simulink model "MPC_sim_noswitch"  (R2017b)
settings: Solver=VariableStepAuto  StartTime=0.0  StopTime=50  FixedStep=0.002  RelTol=1e-3
model workspace (MAT data in the model file):
  ref = Simulink.Parameter
  ref.DataType = 'double'
  ref.Dimensions = [0 0]
libraries: simulink x2, mpclib x1, dspmtrx3 x1
settings Model: Creator=pimwu  LastModifiedBy=pimwu
settings SolverCC: ZeroCrossAlgorithm=Adaptive
settings OptimizationCC: LifeSpan=inf
settings DebuggingCC: SFExecutionAtInitializationDiag=none
settings CodeAppCC: StateflowObjectComments=on

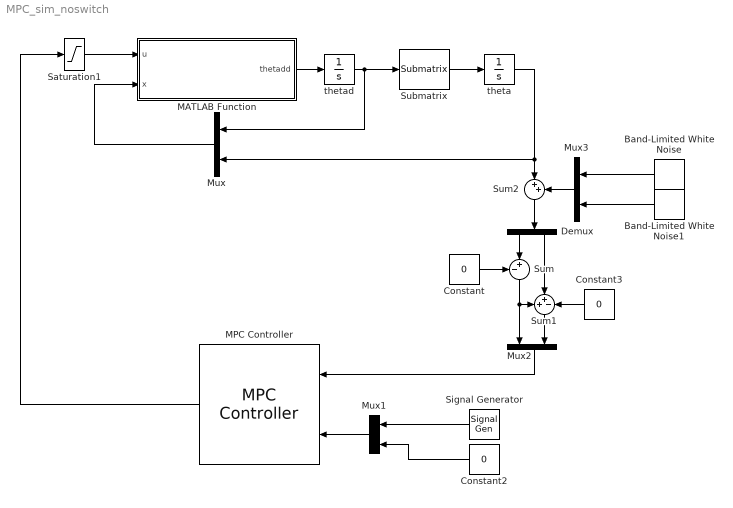
== system MPC_sim_noswitch ==
  Band-Limited White Noise : simulink/Sources/Band-Limited White Noise  Cov=[0.00000001]  Ts=0.002  seed=[23341]
  Band-Limited White Noise1 : simulink/Sources/Band-Limited White Noise  Cov=[0.00000001]  Ts=0.002  seed=[23341]
  Constant : Constant  Value=0
  Constant2 : Constant  Value=0
  Constant3 : Constant  Value=0
  Demux : Demux  Outputs=2
  MATLAB Function : MATLAB Function  TreatAsAtomicUnit=on
  MPC Controller : mpclib/MPC Controller  SCDEnableBlockLinearizationSpecification=on  is_multiple=0  enable_value=0  return_u0=off  ref_from_ws=off  ref_signal_name=[]  ref_preview=off  md_from_ws=off  md_signal_name=[]  md_preview=off  from_project=off  project_file=MPCtask.mat  md_inport=off  mv_inport=off  cost_outport=off  return_sequence=off  return_qpstatus=off  return_state=off  state_inport=off  lims_inport=off  cc_inport=off  ywt_inport=off  is_designfromscratch=0  uwt_inport=off  duwt_inport=off  rhoeps_inport=off  uref_inport=off  n_ts=0.002  n_p=150  n_mv=1  n_md=0  n_ud=0  n_mo=2  n_uo=0  BlockDataType=double  SampleTimeInherited=off  switch_inport=off
  Mux{,1..3} (4 alike) : Mux  Inputs=2
  Saturation1 : Saturate  UpperLimit=1  LowerLimit=-1
  Signal Generator : SignalGenerator  WaveForm=square  Amplitude=0.3  Frequency=1/30
  Submatrix : dspmtrx3/Submatrix  RowSpan=Range of rows  RowStartMode=First  RowStartIndex=1  RowEndMode=Index  RowEndIndex=2  ColSpan=Range of columns  ColStartMode=First  ColStartIndex=1  ColEndMode=Last  ColEndIndex=1
  Sum : Sum  Inputs=-+|
  Sum1 : Sum  Inputs=++-
  Sum2 : Sum  Inputs=|++
  theta : Integrator  InitialCondition=[0.5;0.05]
  thetad : Integrator  InitialCondition=[0 0 0]
  wires:
  MATLAB Function/1(thetadd) -> thetad/1
  thetad/1 -> Submatrix/1, Mux/1
  Submatrix/1 -> theta/1
  Mux/1 -> MATLAB Function/2(x)
  Saturation1/1 -> MATLAB Function/1(u)
  Constant2/1 -> Mux1/2
  MPC Controller/1 -> Saturation1/1
  Constant3/1 -> Sum1/3
  Sum/1 -> Sum1/1, Mux2/1
  Sum1/1 -> Mux2/2
  Constant/1 -> Sum/1
  Demux/2 -> Sum1/2
  Demux/1 -> Sum/2
  theta/1 -> Sum2/1, Mux/2
  Mux3/1 -> Sum2/2
  Band-Limited White Noise/1 -> Mux3/1
  Band-Limited White Noise1/1 -> Mux3/2
  Mux2/1 -> MPC Controller/1
  Mux1/1 -> MPC Controller/2
  Sum2/1 -> Demux/1
  Signal Generator/1 -> Mux1/1

== matlab function MPC_sim_noswitch/MATLAB Function ==
  data: u input; x input; thetadd output
function thetadd = nonlinsim(u,x)
theta1  = x(4);
theta2  = x(5);
theta1d = x(1);
theta2d = x(2);
ii      = x(3);
par =     [0.107001615392530   0.165343973632010   0.040783104942133   0.046364080778153   0.000051655820835   0.048856187724916   0.049137116812930   1.636038234993470   0.000031810472615   1.827977549139487   0.000008590269497   0.006045619229031   3.032790298604742   0.098524631245120   1.049678153165582];

%Define parameters
L1 = par(1);m1 = par(2);m2 = par(3); I1 = par(4); I2 = par(5);
c1 = par(6); c2 = par(7); 
b1 = par(8); b2 = par(9);  Bc1 = par(10); Bc2 = par(11);
 L = par(12); Kt = par(13); R = par(14); Kv = par(15);
g = 9.81;
M = -7;
%Input
Tau = u;%interp1(u.Time,u.Data,t);
ddx = zeros(3,1);
% dx(1) = x(3);
% dx(2) = x(4);
ddx(1) = (3*I2*Kt*ii - 2*Bc2*I2*atan(500*theta1d - 500*theta2d) - 2*Bc1*I2*atan(500*theta1d) - 3*I2*b1*theta1d - 3*I2*b2*theta1d + 3*I2*b2*theta2d - 2*Bc1*c2^2*m2*atan(500*theta1d) - 4*Bc2*c2^2*m2*atan(500*theta1d - 500*theta2d) + 3*Kt*c2^2*ii*m2 - 3*b1*c2^2*m2*theta1d - 6*b2*c2^2*m2*theta1d + 6*b2*c2^2*m2*theta2d + 3*L1*c2^2*g*m2^2*sin(theta1) + 3*I2*c2*g*m2*sin(theta1 + theta2) + 3*I2*L1*g*m2*sin(theta1) + 3*I2*c1*g*m1*sin(theta1) + 3*L1*c2^3*m2^2*theta1d^2*sin(theta2) + 3*L1*c2^3*m2^2*theta2d^2*sin(theta2) + 6*L1*c2^3*m2^2*theta1d*theta2d*sin(theta2) - 3*L1*b2*c2*m2*theta1d*cos(theta2) + 3*L1*b2*c2*m2*theta2d*cos(theta2) + 3*L1^2*c2^2*m2^2*theta1d^2*cos(theta2)*sin(theta2) - 3*L1*c2^2*g*m2^2*sin(theta1 + theta2)*cos(theta2) + 3*I2*L1*c2*m2*theta2d^2*sin(theta2) + 3*c1*c2^2*g*m1*m2*sin(theta1) - 2*Bc2*L1*c2*m2*atan(500*theta1d - 500*theta2d)*cos(theta2) + 6*I2*L1*c2*m2*theta1d*theta2d*sin(theta2))/(3*(I1*I2 + L1^2*c2^2*m2^2 + I2*L1^2*m2 + I1*c2^2*m2 + I2*c2^2*m2 - L1^2*c2^2*m2^2*cos(theta2)^2 + 2*I2*L1*c2*m2*cos(theta2)));
ddx(2) =  -(3*I1*b2*theta2d - 3*I1*b2*theta1d - 2*Bc2*I1*atan(500*theta1d - 500*theta2d) - 2*Bc1*c2^2*m2*atan(500*theta1d) - 2*Bc2*L1^2*m2*atan(500*theta1d - 500*theta2d) - 4*Bc2*c2^2*m2*atan(500*theta1d - 500*theta2d) + 3*Kt*c2^2*ii*m2 - 3*L1^2*b2*m2*theta1d + 3*L1^2*b2*m2*theta2d - 3*b1*c2^2*m2*theta1d - 6*b2*c2^2*m2*theta1d + 6*b2*c2^2*m2*theta2d - 3*L1^2*c2*g*m2^2*sin(theta1 + theta2) + 3*L1*c2^2*g*m2^2*sin(theta1) - 3*I1*c2*g*m2*sin(theta1 + theta2) + 3*L1*c2^3*m2^2*theta1d^2*sin(theta2) + 3*L1^3*c2*m2^2*theta1d^2*sin(theta2) + 3*L1*c2^3*m2^2*theta2d^2*sin(theta2) + 3*Kt*L1*c2*ii*m2*cos(theta2) + 6*L1*c2^3*m2^2*theta1d*theta2d*sin(theta2) - 3*L1*b1*c2*m2*theta1d*cos(theta2) - 9*L1*b2*c2*m2*theta1d*cos(theta2) + 9*L1*b2*c2*m2*theta2d*cos(theta2) + 6*L1^2*c2^2*m2^2*theta1d^2*cos(theta2)*sin(theta2) + 3*L1^2*c2^2*m2^2*theta2d^2*cos(theta2)*sin(theta2) - 3*L1*c2^2*g*m2^2*sin(theta1 + theta2)*cos(theta2) + 3*L1^2*c2*g*m2^2*cos(theta2)*sin(theta1) + 3*I1*L1*c2*m2*theta1d^2*sin(theta2) + 3*c1*c2^2*g*m1*m2*sin(theta1) - 2*Bc1*L1*c2*m2*atan(500*theta1d)*cos(theta2) - 6*Bc2*L1*c2*m2*atan(500*theta1d - 500*theta2d)*cos(theta2) + 6*L1^2*c2^2*m2^2*theta1d*theta2d*cos(theta2)*sin(theta2) + 3*L1*c1*c2*g*m1*m2*cos(theta2)*sin(theta1))/(3*(I1*I2 + L1^2*c2^2*m2^2 + I2*L1^2*m2 + I1*c2^2*m2 + I2*c2^2*m2 - L1^2*c2^2*m2^2*cos(theta2)^2 + 2*I2*L1*c2*m2*cos(theta2)));
ddx(3) = -(R*ii - M*Tau + Kv*theta1d)/L;
% dx = dx';

end
